simulink model "hexa_tilted_SMC"  (R2023a)
settings: Solver=ode4  StartTime=0.0  StopTime=tf  FixedStep=0.01  RelTol=1e-3
model workspace (MAT data in the model file):
  tf = Simulink.Parameter
  tf.Value = 60
  tf.DataType = 'auto'
  tf.Complexity = 'real'
  tf.Dimensions = [1 1]
  tray1 = [0  0  0  0  0  0; 0  0  0  0  0  0; 0  5  2.5  5  2.5  0; 0  0  0  0  0  0; 0  0  0  0  0  0; 0  0  0  0  0  0]
  tray2 = [0  2  2  -2  -2  0; 0  0  -2  -2  2  0; 0  5  2.5  5  2.5  0; 0  0  0  0  0  0; 0  0  0  0  0  0; 0  0  0  0  0  0]
  tray3 = [0  2  2  -2  -2  0; 0  0  -2  -2  2  0; 0  5  2.5  5  2.5  0; 0  0  0  0  0  0; 0  0  0  0  0  0; 0  0  0.785  1.57  0.785  0]
  tray4 = [0  2  2  -2  -2  0; 0  0  -2  -2  2  0; 0  5  2.5  5  2.5  0; 0  0.15  0.15  0.15  0.15  0; 0  0  0  0  0  0; 0  0  0.785  1.57  0.785  0]
  tray5 = [0  0  0  0  0  0; 0  0  0  0  0  0; 0  5  2.5  5  2.5  0; 0  0.15  0.15  0  0  0; 0  0  0.15  0.15  0  0; 0  0  0  0  0  0]
libraries: robotcorelib x1
settings Model: Creator=adan  LastModifiedBy=Adan Daniel
settings OptimizationCC: ReuseModelBlockBuffer=off

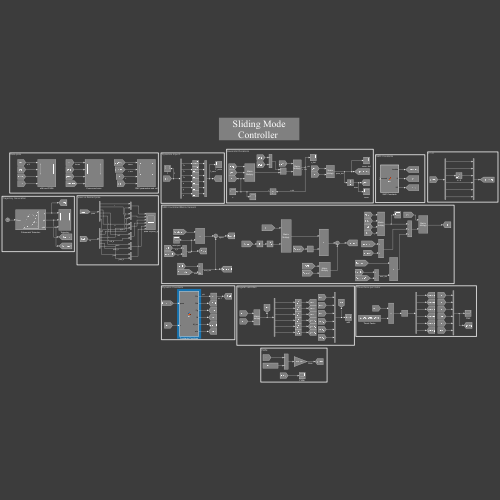
[thumbnail: Simulink's stored preview of the top-level diagram]
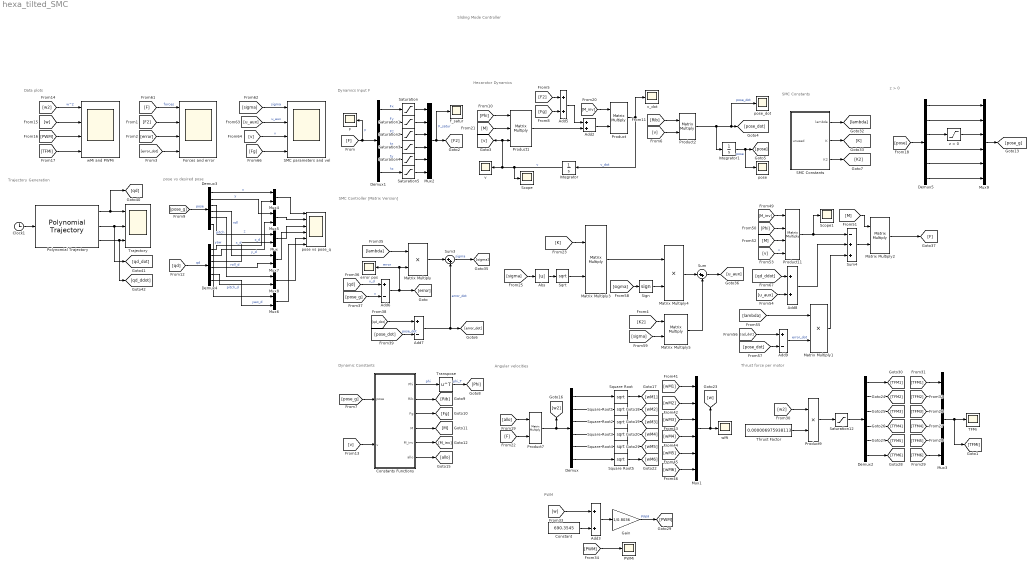
== system hexa_tilted_SMC ==
  note: Sliding Mode Controller
  note: z > 0
  note: SMC Controller [Matrix Version]
  note: pose vs desired pose
  note: Trajectory Generation
  note: Dynamic Constants
  note: Data plots
  note: SMC Constants
  note: PWM
  note: Angular velocities
  note: Thrust force per motor
  note: Hexarotor Dynamics
  note: Dynamics Input F
  Abs : Abs  SaturateOnIntegerOverflow=off
  Add{2..3,5,8} (4 alike) : Sum
  Add6 : Sum  Inputs=+-
  Add7 : Sum  Inputs=+-
  Add9 : Sum  Inputs=+-
  Clock1 : Clock
  Constant : Constant  Value=690.3545
  Constants Functions : MATLAB Function  TreatAsAtomicUnit=on
  Demux{,1..5} (6 alike) : Demux  Outputs=6
  F : Scope
  F_satur : Scope
  Forces and error : Scope  NumInputPorts=4
  Gain : Gain  Gain=1/0.8036
  Integrator : Integrator  InitialCondition=[0; 0; 0; 0; 0; 0]
  Integrator1 : Integrator  InitialCondition=[0; 0; 0; 0; 0; 0]
  Matrix Multiply : Product
  Matrix Multiply1 : Product
  Matrix Multiply2 : Product  Multiplication=Matrix(*)
  Matrix Multiply3 : Product  Multiplication=Matrix(*)
  Matrix Multiply4 : Product
  Matrix Multiply5 : Product  Multiplication=Matrix(*)
  Mux{,4..8} (6 alike) : Mux  Inputs=2
  Mux{1..3,9} (4 alike) : Mux  Inputs=6
  PWMi : Scope
  Polynomial Trajectory : robotcorelib/Polynomial Trajectory  WaypointSource=Internal  Waypoints=tray3  TimePoints=[ 0, 12, 24, 35, 48, tf ]  TimeInterval=[ 1, 4 ]  Method=Cubic Polynomial  ParameterSource=Internal  VelocityBoundaryCondition=zeros( 6, 6 )  AccelerationBoundaryCondition=zeros( 2, 5 )  SimulateUsing=Interpreted execution
  Product : Product  Multiplication=Matrix(*)
  Product1 : Product  Inputs=3  Multiplication=Matrix(*)
  Product11 : Product  Inputs=4  Multiplication=Matrix(*)
  Product2 : Product  Multiplication=Matrix(*)
  Product7 : Product  Multiplication=Matrix(*)
  Product9 : Product
  SMC Constants : MATLAB Function  TreatAsAtomicUnit=on
  SMC parameters and vel : Scope  NumInputPorts=4
  Saturation : Saturate  UpperLimit=6  LowerLimit=-6
  Saturation1 : Saturate  UpperLimit=6  LowerLimit=-6
  Saturation12 : Saturate  UpperLimit=818608.7529  LowerLimit=0
  Saturation2 : Saturate  UpperLimit=5.8*6  LowerLimit=0
  Saturation3 : Saturate
  Saturation4 : Saturate
  Saturation5 : Saturate
  Scope : Scope
  Scope1 : Scope
  Sign : Signum
  Sqrt : Sqrt
  Square Root{,1..5} (6 alike) : Sqrt
  Sum : Sum  Inputs=|++
  Sum3 : Sum  Inputs=|++
  Sum4 : Sum  Inputs=-++
  TFMi : Scope
  Thrust Factor : Constant  Value=0.000006975938113
  Trajectory : Scope  NumInputPorts=3
  Transpose : Math  Operator=transpose
  error pos : Scope
  pose : Scope
  pose vs pose_q : Scope  NumInputPorts=6
  pose_dot : Scope
  v : Scope
  v_dot : Scope
  wMi : Scope
  wMi and PWMi : Scope  NumInputPorts=4
  z > 0 : Saturate  UpperLimit=100  LowerLimit=0
  wires:
  Saturation/1 -> Mux2/1
  Saturation1/1 -> Mux2/2
  Saturation4/1 -> Mux2/5
  Saturation3/1 -> Mux2/4
  Demux1/6 -> Saturation5/1  "tz"
  Demux1/3 -> Saturation2/1  "Fz"
  [F] -> F/1, Demux1/1  "F"
  Saturation5/1 -> Mux2/6
  Demux1/2 -> Saturation1/1  "Fy"
  Demux1/1 -> Saturation/1  "Fx"
  Demux1/5 -> Saturation4/1  "ty"
  Demux1/4 -> Saturation3/1  "tx"
  Saturation2/1 -> Mux2/3
  Mux2/1 -> [F2], F_satur/1  "F_satur"
  [M] -> Product1/2
  [v] -> Product2/2
  [M_inv] -> Product/1
  Add2/1 -> Product/2
  Product/1 -> v_dot/1, Integrator/1  "v_dot"
  [Rib] -> Product2/1
  Product2/1 -> Integrator1/1, pose_dot/1, [pose_dot]  "pose_dot"
  [Phi] -> Product1/1
  Product1/1 -> Add2/2
  Integrator1/1 -> pose/1, [pose]  "pose"
  Integrator/1 -> Scope/1, v/1, [v], Product1/3  "v"
  [Fg] -> Add5/2
  Add5/1 -> Add2/1
  [TFM6] -> Mux3/6
  Demux2/2 -> [TFM2]
  [TFM3] -> Mux3/3
  Demux2/6 -> [TFM6]
  [TFM5] -> Mux3/5
  Saturation12/1 -> Demux2/1
  [TFM2] -> Mux3/2
  [TFM1] -> Mux3/1
  Demux2/5 -> [TFM5]
  Demux2/4 -> [TFM4]
  Product9/1 -> Saturation12/1
  Demux2/1 -> [TFM1]
  Thrust Factor/1 -> Product9/2
  Demux2/3 -> [TFM3]
  [w2] -> Product9/1
  [TFM4] -> Mux3/4
  [wM1] -> Mux1/1
  Square Root/1 -> [wM1]
  [wM5] -> Mux1/5
  Square Root5/1 -> [wM6]
  Square Root3/1 -> [wM4]
  [F] -> Product7/2
  [allo] -> Product7/1
  [wM2] -> Mux1/2
  Demux/6 -> Square Root5/1
  Demux/5 -> Square Root4/1
  Square Root1/1 -> [wM2]
  [wM3] -> Mux1/3
  Square Root2/1 -> [wM3]
  Demux/4 -> Square Root3/1
  Demux/2 -> Square Root1/1
  Demux/3 -> Square Root2/1
  Square Root4/1 -> [wM5]
  Product7/1 -> [w2], Demux/1
  Demux/1 -> Square Root/1
  [wM4] -> Mux1/4
  Mux1/1 -> [w], wMi/1
  [wM6] -> Mux1/6
  Mux3/1 -> [TFMi], TFMi/1
  Constant/1 -> Add3/2
  [PWM] -> PWMi/1
  [w] -> Add3/1
  Gain/1 -> [PWM]  "PWM"
  Add3/1 -> Gain/1
  SMC Constants/1(lambda) -> [lambda]
  SMC Constants/2(K) -> [K]
  [u_aux] -> SMC parameters and vel/2  "u_aux"
  [v] -> SMC parameters and vel/3  "v"
  [sigma] -> SMC parameters and vel/1  "sigma"
  [F2] -> Add5/1
  [Fg] -> SMC parameters and vel/4
  [pose_g] -> Constants Functions/1(pose)
  [v] -> Constants Functions/2(v)
  Constants Functions/6(allo) -> [allo]
  Constants Functions/3(Fg) -> [Fg]
  Constants Functions/4(M) -> [M]
  Constants Functions/1(Phi) -> Transpose/1  "phi"
  Constants Functions/2(Rib) -> [Rib]
  Transpose/1 -> [Phi]  "phi_T"
  Constants Functions/5(M_inv) -> [M_inv]
  Clock1/1 -> Polynomial Trajectory/1
  Polynomial Trajectory/2 -> [qd_dot], Trajectory/2
  Polynomial Trajectory/3 -> [qd_ddot], Trajectory/3
  Demux4/3 -> Mux/2  "z_d"
  Demux3/6 -> Mux6/1  "yaw"
  Demux3/2 -> Mux5/1  "y"
  Demux3/4 -> Mux7/1  "roll"
  Mux/1 -> pose vs pose_q/3
  [qd] -> Demux4/1  "qd"
  [pose_g] -> Demux3/1  "pose"
  Demux3/1 -> Mux4/1  "x"
  Demux4/6 -> Mux6/2  "yaw_d"
  Mux5/1 -> pose vs pose_q/2
  Demux4/2 -> Mux5/2  "y_d"
  Demux4/5 -> Mux8/2  "pitch_d"
  Mux4/1 -> pose vs pose_q/1
  Demux4/1 -> Mux4/2  "x_d"
  Demux3/5 -> Mux8/1  "pitch"
  Demux3/3 -> Mux/1  "z"
  Demux4/4 -> Mux7/2  "roll_d"
  Polynomial Trajectory/1 -> [qd], Trajectory/1
  [F] -> Forces and error/1  "forces"
  [F2] -> Forces and error/2
  [error] -> Forces and error/3
  [error_dot] -> Forces and error/4
  [TFMi] -> wMi and PWMi/4
  [w] -> wMi and PWMi/2
  [w2] -> wMi and PWMi/1  "w^2"
  [PWM] -> wMi and PWMi/3
  SMC Constants/3(K2) -> [K2]
  Mux6/1 -> pose vs pose_q/6
  Mux7/1 -> pose vs pose_q/4
  Mux8/1 -> pose vs pose_q/5
  [M] -> Product11/3
  Add8/1 -> Sum4/2
  [lambda] -> Matrix Multiply/1
  [K] -> Matrix Multiply3/1
  [u_aux] -> Add8/2
  [pose_dot] -> Add7/2  "pose_dot"
  [K2] -> Matrix Multiply5/1
  Matrix Multiply1/1 -> Sum4/3
  [sigma] -> Matrix Multiply5/2
  Matrix Multiply/1 -> Sum3/1
  [pose_g] -> Add6/2  "x"
  [M_inv] -> Product11/1
  [qd_dot] -> Add7/1
  Matrix Multiply2/1 -> [F]
  Sum4/1 -> Matrix Multiply2/2
  Add9/1 -> Matrix Multiply1/2  "error_dot"
  [sigma] -> Abs/1
  Sqrt/1 -> Matrix Multiply3/2
  Matrix Multiply3/1 -> Matrix Multiply4/1
  Matrix Multiply5/1 -> Sum/2
  Sum3/1 -> [sigma]  "sigma"
  Product11/1 -> Scope1/1, Sum4/1
  [qd] -> Add6/1  "x_d"
  [v] -> Product11/4  "v"
  Sum/1 -> [u_aux]
  [sigma] -> Sign/1
  [lambda] -> Matrix Multiply1/1
  Add6/1 -> [error], Matrix Multiply/2, error pos/1  "error"
  [Phi] -> Product11/2
  Sign/1 -> Matrix Multiply4/2
  [pose_dot] -> Add9/2
  Matrix Multiply4/1 -> Sum/1
  [qd_ddot] -> Add8/1
  [qd_dot] -> Add9/1
  [M] -> Matrix Multiply2/1
  Add7/1 -> [error_dot], Sum3/2  "error_dot"
  Abs/1 -> Sqrt/1
  Mux9/1 -> [pose_g]
  Demux5/5 -> Mux9/5
  Demux5/4 -> Mux9/4
  [pose] -> Demux5/1
  Demux5/3 -> z > 0/1
  Demux5/2 -> Mux9/2
  z > 0/1 -> Mux9/3
  Demux5/1 -> Mux9/1
  Demux5/6 -> Mux9/6

== matlab function hexa_tilted_SMC/SMC Constants ==
  data: unused input; lambda output; K output; K2 output
function [lambda, K, K2] = fcn(~)

% valores de lambda > 0
lambda = [0.25; 0.25; 10; 0.25; 0.25; 0.25];

% valores de K > 0
%K = [7.5; 7.5; 15; 5; 5; 5];

K = [7.5, 0, 0, 0, 0, 0;
     0, 7.5, 0, 0, 0, 0;
     0, 0, 15, 0, 0, 0;
     0, 0, 0, 5, 0, 0;
     0, 0, 0, 0, 5, 0;
     0, 0, 0, 0, 0, 5];

K2 = [0, 0, 0, 0, 0, 0;
     0, 0, 0, 0, 0, 0;
     0, 0, 0.1, 0, 0, 0;
     0, 0, 0, 5, 0, 0;
     0, 0, 0, 0, 5, 0;
     0, 0, 0, 0, 0, 5];

== matlab function hexa_tilted_SMC/Constants Functions ==
  data: Phi output; Rib output; Fg output; pose input; M output; M_inv output; allo output; v input
function [Phi, Rib, Fg, M, M_inv, allo] = fcn(pose, v)

%% system constants
pi = 3.141592;
m = 2.0; %5 mass 2.2 kg
l = 0.25; % length m
g = 9.81; % gravity m/s²
Jxx =  24778420.82/(1000*1000000); % kg m²
Jyy = 42217933.96/(1000*1000000); % kg m²
Jzz = 23948304.24/(1000*1000000); % kg m²
kT = 0.000006975938113;
kQ = 0.000118290418538;

%% Phi matrix calculation
uu = v(1);
vv = v(2);
ww = v(3);
pp = v(4);
qq = v(5);
rr = v(6);


Phi = [0, -rr, qq, 0, -ww, vv;
        rr, 0, -pp , ww, 0, -uu;
        -qq, pp, 0,  -vv, uu, 0;
        0, 0, 0, 0, -rr, qq; 
        0, 0, 0, rr, 0, -pp;
        0, 0, 0, -qq, pp, 0];

%% Rib matrix calculation

roll = pose(4);
pitch = pose(5);
yaw = pose(6);

Rib = [cos(yaw)*cos(pitch), -cos(roll)*sin(yaw) + cos(yaw)*sin(roll)*sin(pitch), sin(roll)*sin(yaw) + cos(roll)*cos(yaw)*sin(pitch), 0, 0, 0;
       cos(pitch)*sin(yaw), cos(roll)*cos(yaw) + sin(yaw)*sin(pitch)*sin(roll), -cos(yaw)*sin(roll) + sin(yaw)*sin(pitch)*cos(roll), 0, 0, 0;
       -sin(pitch), cos(pitch)*sin(roll), cos(pitch)*cos(roll), 0, 0, 0;
       0, 0, 0, 1, sin(roll)*tan(pitch), cos(roll)*tan(pitch);
       0, 0, 0, 0, cos(roll), -sin(roll);
       0, 0, 0, 0, sin(roll)/cos(pitch), cos(roll)/cos(pitch)];

%% Fg matrix calculation

Fg = [m*g*sin(pitch);
      -m*g*cos(pitch)*sin(roll);
      -m*g*cos(pitch)*cos(roll);
      0;
      0;
      0];

M = [m, 0, 0, 0, 0, 0;
    0, m, 0, 0, 0, 0;
    0, 0, m, 0, 0, 0;
    0, 0, 0, Jxx, 0, 0;
    0, 0, 0, 0, Jyy, 0;
    0, 0, 0, 0, 0, Jzz];

M_inv = inv(M);

alpha = [pi/6; -pi/6; -pi/2; -5*pi/6; 5*pi/6; pi/2];

varphi = pi/9;

%% tilted rotors matrix allocation

m11 = -kT*cos(alpha(1))*sin(varphi);
m21 = kT*sin(alpha(1))*sin(varphi);
m31 = kT*cos(varphi);
m41 = cos(alpha(1))*(l*kT*cos(varphi) - kQ*sin(varphi));
m51 = sin(alpha(1))*(-l*kT*cos(varphi) + kQ*sin(varphi));
m61 = l*kT*sin(varphi) + kQ*cos(varphi);

m12 = kT*cos(alpha(2))*sin(varphi);
m22 = -kT*sin(alpha(2))*sin(varphi);
m32 = m31;
m42 = cos(alpha(2))*(l*kT*cos(varphi) - kQ*sin(varphi));
m52 = sin(alpha(2))*(-l*kT*cos(varphi) + kQ*sin(varphi));
m62 = -l*kT*sin(varphi) - kQ*cos(varphi);

m13 = kT*cos(alpha(3))*sin(varphi);
m23 = kT*sin(alpha(3))*sin(varphi);
m33 = m31;
m43 = cos(alpha(3))*(l*kT*cos(varphi) + kQ*sin(varphi));
m53 = sin(alpha(3))*(-l*kT*cos(varphi) + kQ*sin(varphi));
m63 = l*kT*sin(varphi) + kQ*cos(varphi);

m14 = kT*cos(alpha(4))*sin(varphi);
m24 = -kT*sin(alpha(4))*sin(varphi);
m34 = m31;
m44 = cos(alpha(4))*(l*kT*cos(varphi) - kQ*sin(varphi));
m54 = sin(alpha(4))*(-l*kT*cos(varphi) + kQ*sin(varphi));
m64 = -l*kT*sin(varphi) - kQ*cos(varphi);

m15 = -kT*cos(alpha(5))*sin(varphi);
m25 = kT*sin(alpha(5))*sin(varphi);
m35 = m31;
m45 = cos(alpha(5))*(l*kT*cos(varphi) - kQ*sin(varphi));
m55 = sin(alpha(5))*(-l*kT*cos(varphi) + kQ*sin(varphi));
m65 = l*kT*sin(varphi) + kQ*cos(varphi);

m16 = kT*cos(alpha(6))*sin(varphi);
m26 = -kT*sin(alpha(6))*sin(varphi);
m36 = m31;
m46 = cos(alpha(6))*(l*kT*cos(varphi) + kQ*sin(varphi));
m56 = sin(alpha(6))*(-l*kT*cos(varphi) + kQ*sin(varphi));
m66 = -l*kT*sin(varphi) - kQ*cos(varphi);

allo = [m11, m12, m13, m14, m15, m16;
        m21, m22, m23, m24, m25, m26;
        m31, m32, m33, m34, m35, m36;
        m41, m42, m43, m44, m45, m46;
        m51, m52, m53, m54, m55, m56;
        m61, m62, m63, m64, m65, m66];

allo = inv(allo);
